simulink model "growth_system_OD"  (R2023a)
settings: Solver=VariableStepAuto  StartTime=0.0  StopTime=1000  RelTol=1e-3
settings Model: Creator=Lucca  LastModifiedBy=Lucca

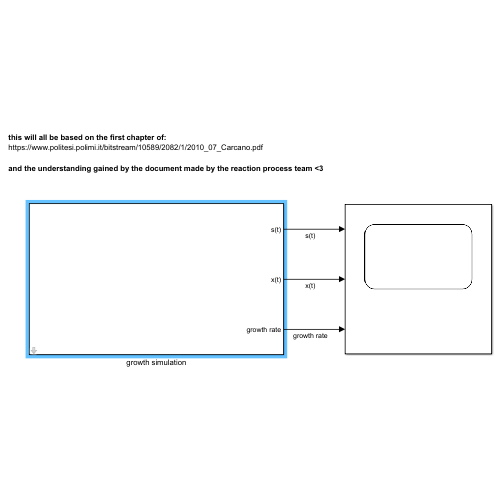
[thumbnail: Simulink's stored preview of the top-level diagram]
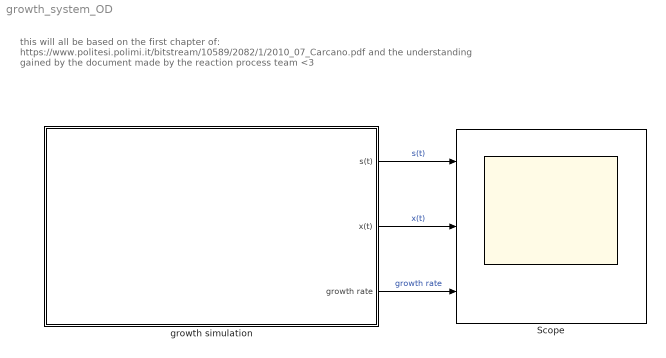
== system growth_system_OD ==
  note: this will all be based on the first chapter of:
      | https://www.politesi.polimi.it/bitstream/10589/2082/1/2010_07_Carcano.pdf
      |
      | and the understanding gained by the document made by the reaction process team <3
  Scope : Scope  NumInputPorts=3
  growth simulation : Subsystem  mask{y=0.4, x0=1.5, s0=2, max_gr=0.0271, Ks=0.0376, V=0.025, vin=0, vout=0, C_s0=1}
      mask prompts: y "growth yield"; x0 "initial number of cells"; s0 "initial conc of substrate (kg)"; max_gr "max growth rate (s^-1)"; Ks "half-maximum constant (kg/L)"; V "working volume (L)"; vin "inflow of liquid (L/s)"; vout "outflow of liquid (L/s)"; C_s0 "Concentration of susbstrate in premade solution (kg/L)"
  wires:
  growth simulation/1(s(t)) -> Scope/1  "s(t)"
  growth simulation/2(x(t)) -> Scope/2  "x(t)"
  growth simulation/3(growth rate) -> Scope/3  "growth rate"

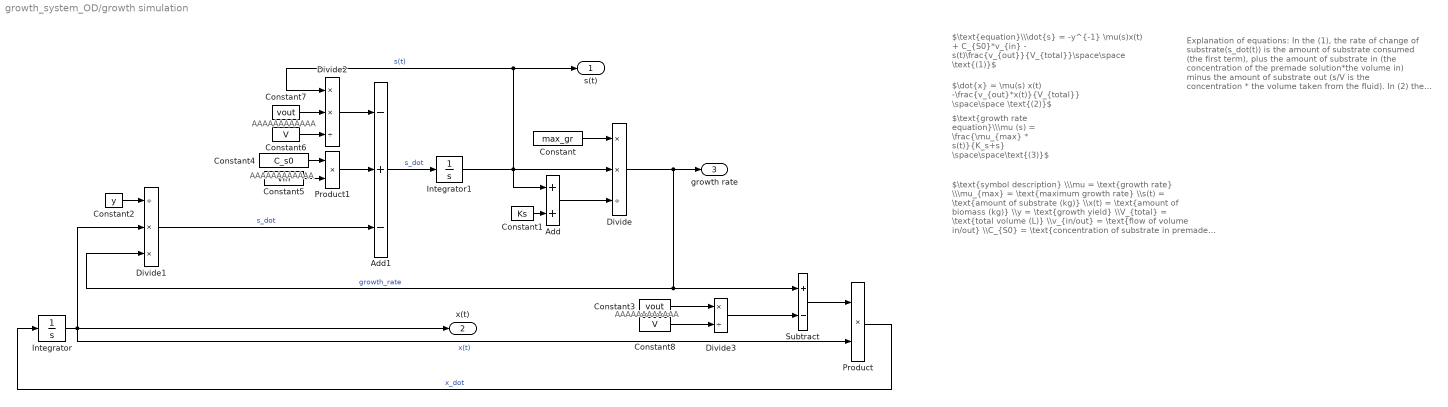
== system growth_system_OD/growth simulation ==
  note: Explanation of equations:
      |
      | In the (1), the rate of change of substrate(s_dot(t)) is the amount of substrate consumed (the first term), plus the amount of substrate in (the concentration of the premade solution*the volume in) minus the amount of substrate out (s/V is the concentration * the volume taken from the fluid).
      |
      | In (2) the first term describes the growth of biomass over time x(t) minus the amount of biomass lost when some volume is flushed out.
      |
      | (3) is the Monod growth equation to describe the growht of biomass.
  note: AAAAAAAAAAAA
  note: $\text{symbol description} \\\mu = \text{growth rate} \\\mu_{max} = \text{maximum growth rate} \\s(t) = \text{amount of substrate (kg)} \\x(t) = \text{amount of biomass (kg)} \\y = \text{growth yield} \\V_{total} = \text{total volume (L)} \\v_{in/out} = \text{flow of volume in/out} \\C_{S0} = \text{concentration of substrate in premade solution} \\C_{S} = \text{concentration of substrate in the media} \\K_{s} = \text{half-maximum constant}$
      | All values are considered using SI units (kg,L,s), so even if not shown the units will be in these values (e.g. Cs [kg/L)]
      |
      | OBS ANY CONSTANTS WITH YELLOW MARKER ON THE SIDE SHOULD BE CHANGED WHEN THE INTEGRATED MODEL IS CREATED
  note: $\text{growth rate equation}\\\mu (s) = \frac{\mu_{max} * s(t)}{K_s+s} \space\space\text{(3)}$
  note: $\text{equation}\\\dot{s} = -y^{-1} \mu(s)x(t) + C_{S0}*v_{in} - s(t)\frac{v_{out}}{V_{total}}\space\space \text{(1)}$
  note: $\dot{x} = \mu(s) x(t) -\frac{v_{out}*x(t)}{V_{total}} \space\space \text{(2)}$
  note: AAAAAAAAAAAA
  note: AAAAAAAAAAAA
  Add : Sum
  Add1 : Sum  Inputs=-+-
  Constant : Constant  Value=max_gr
  Constant1 : Constant  Value=Ks
  Constant2 : Constant  Value=y
  Constant3 : Constant  Value=vout
  Constant4 : Constant  Value=C_s0
  Constant5 : Constant  Value=vin
  Constant6 : Constant  Value=V
  Constant7 : Constant  Value=vout
  Constant8 : Constant  Value=V
  Divide : Product  Inputs=**/
  Divide1 : Product  Inputs=/**
  Divide2 : Product  Inputs=**/
  Divide3 : Product  Inputs=*/
  Integrator : Integrator  InitialCondition=x0
  Integrator1 : Integrator  InitialCondition=s0
  Product : Product
  Product1 : Product
  Subtract : Sum  Inputs=+-
  s(t) : Outport
  x(t) : Outport  Port=2
  growth rate : Outport  Port=3
  wires:
  Integrator/1 -> Product/2, x(t)/1, Divide1/2  "x(t)"
  Product/1 -> Integrator/1  "x_dot"
  Integrator1/1 -> Divide2/1, s(t)/1, Divide/2, Add/1  "s(t)"
  Add1/1 -> Integrator1/1  "s_dot"
  Constant/1 -> Divide/1
  Add/1 -> Divide/3
  Constant1/1 -> Add/2
  Divide/1 -> Subtract/1, Divide1/3, growth rate/1  "growth_rate"
  Constant2/1 -> Divide1/1
  Divide3/1 -> Subtract/2
  Subtract/1 -> Product/1
  Divide1/1 -> Add1/3  "s_dot"
  Constant4/1 -> Product1/1
  Product1/1 -> Add1/2
  Constant5/1 -> Product1/2
  Divide2/1 -> Add1/1
  Constant6/1 -> Divide2/3
  Constant7/1 -> Divide2/2
  Constant8/1 -> Divide3/2
  Constant3/1 -> Divide3/1
